simulink model "PID_Controller_Simulink"  (R2023b)
settings: Solver=VariableStepAuto  StartTime=0.0  StopTime=10  RelTol=1e-3
settings Model: Creator=Lenovo  LastModifiedBy=KhyathiB

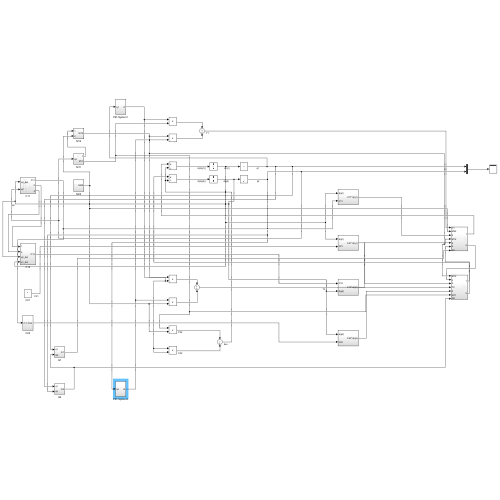
[thumbnail: Simulink's stored preview of the top-level diagram]
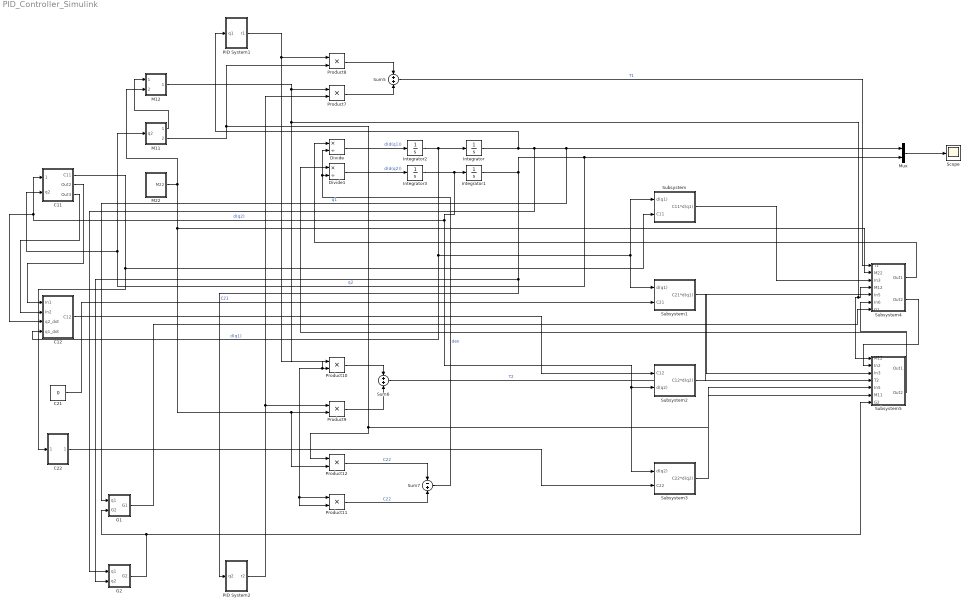
== system PID_Controller_Simulink ==
  C11 : Subsystem
  C12 : Subsystem
  C21 : Constant  Value=0
  C22 : Subsystem
  Divide : Product  Inputs=*/
  Divide1 : Product  Inputs=*/
  G1 : Subsystem
  G2 : Subsystem
  Integrator : Integrator  InitialCondition=0.1
  Integrator1 : Integrator  InitialCondition=0.1
  Integrator2 : Integrator
  Integrator3 : Integrator
  M11 : Subsystem
  M12 : Subsystem
  M22 : Subsystem
  Mux : Mux  Inputs=2
  PID System1 : Subsystem
  PID System2 : Subsystem
  Product{7..12} (6 alike) : Product
  Scope : Scope
  Subsystem : Subsystem
  Subsystem1 : Subsystem
  Subsystem2 : Subsystem
  Subsystem3 : Subsystem
  Subsystem4 : Subsystem
  Subsystem5 : Subsystem
  Sum5 : Sum
  Sum6 : Sum
  Sum7 : Sum  Inputs=-+
  wires:
  Mux/1 -> Scope/1
  Integrator/1 -> G2/1(q1), G1/1(q1), Mux/1, PID System1/1(q1)  "q1"
  Integrator1/1 -> G2/2(q2), PID System2/1(q2), C11/2(q2), M11/1(q2), Mux/2  "q2"
  Integrator2/1 -> Integrator/1, C12/4(q1_dot), Subsystem1/1(d(q1)), Subsystem/1(d(q1))  "d(q1)"
  Integrator3/1 -> Subsystem3/1(d(q2)), Subsystem2/2(d(q2)), C12/3(q2_dot), C11/1(q2_dot), Integrator1/1  "d(q2)"
  Divide1/1 -> Integrator3/1  "d(d(q2))"
  Divide/1 -> Integrator2/1  "d(d(q1))"
  PID System2/1(r2) -> Product7/2, Product9/1
  PID System1/1(r1) -> Product10/1, Product8/1
  Product8/1 -> Sum5/1
  Product7/1 -> Sum5/2
  Product9/1 -> Sum6/2
  Product10/1 -> Sum6/1
  Product12/1 -> Sum7/1  "C22"
  Product11/1 -> Sum7/2  "C22"
  Sum7/1 -> Divide/2, Divide1/2  "den"
  C21/1 -> Subsystem1/2(C21)  "C21"
  Sum5/1 -> Subsystem4/1(T1)  "T1"
  Subsystem/1(C11*d(q1)) -> Subsystem4/3(In3)
  Subsystem2/1(C12*d(q2)) -> Subsystem4/5(In5)
  Subsystem4/1(Out1) -> Divide/1
  Subsystem4/2(Out2) -> Subsystem5/2(In2)
  Subsystem1/1(C21*d(q1)) -> Subsystem5/3(In3)
  Sum6/1 -> Subsystem5/4(T2)  "T2"
  Subsystem3/1(C22*d(q2)) -> Subsystem5/5(In5)
  Subsystem5/1(Out1) -> Divide1/1
  Subsystem5/2(Out2) -> Subsystem4/6(In6)
  M22/1(M22) -> M12/2(In2), Subsystem4/2(M22), Product9/2, Product12/2
  M11/2(M11) -> Product8/2, Product12/1, Subsystem5/6(M11)
  M12/1(M12) -> Product11/1, Product11/2, Product10/2, Subsystem4/4(M12), Subsystem5/1(M12), Product7/1
  M11/1(Out1) -> M12/1(In1)
  C11/1(C11) -> C22/1(C11), Subsystem/2(C11)
  C11/2(Out2) -> C12/1(In1)
  C11/3(Out3) -> C12/2(In2)
  C12/1(C12) -> Subsystem2/1(C12)
  C22/1(C22) -> Subsystem3/2(C22)
  G2/1(G2) -> G1/2(G2), Subsystem5/7(G2)
  G1/1(G1) -> Subsystem4/7(G1)

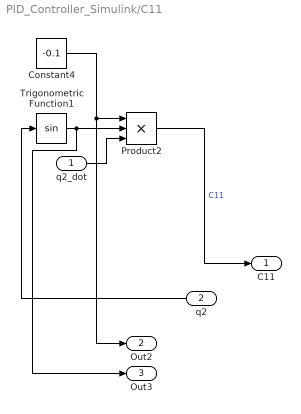
== system PID_Controller_Simulink/C11 ==
  q2_dot : Inport
  q2 : Inport  Port=2
  Constant4 : Constant  Value=-0.1
  Product2 : Product  Inputs=3
  Trigonometric Function1 : Trigonometry
  C11 : Outport
  Out2 : Outport  Port=2
  Out3 : Outport  Port=3
  wires:
  Constant4/1 -> Out2/1, Product2/1
  Trigonometric Function1/1 -> Out3/1, Product2/2
  q2/1 -> Trigonometric Function1/1
  Product2/1 -> C11/1  "C11"
  q2_dot/1 -> Product2/3

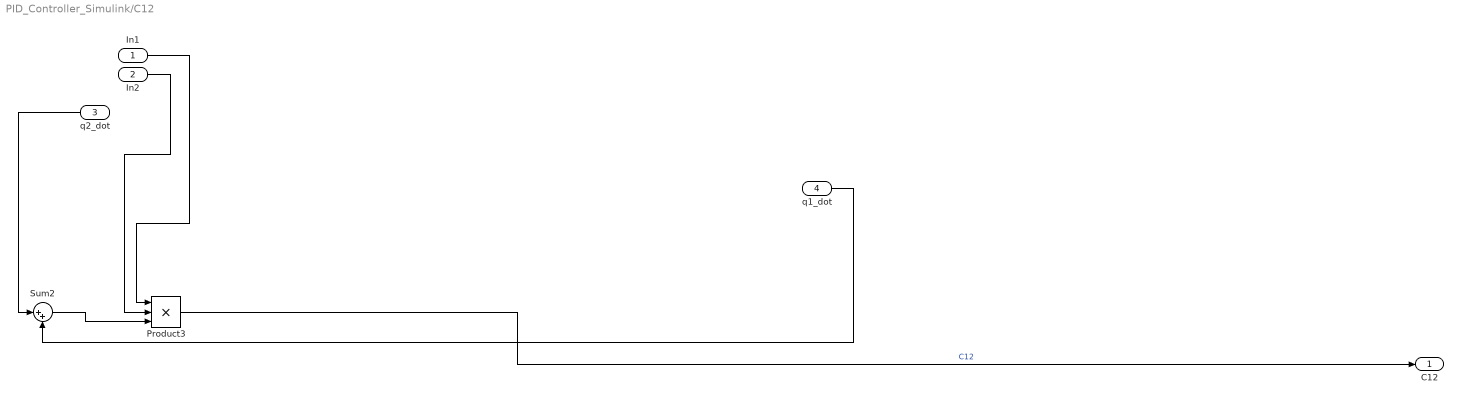
== system PID_Controller_Simulink/C12 ==
  In1 : Inport
  In2 : Inport  Port=2
  q2_dot : Inport  Port=3
  q1_dot : Inport  Port=4
  Product3 : Product  Inputs=3
  Sum2 : Sum  Inputs=|++
  C12 : Outport
  wires:
  In2/1 -> Product3/2
  Sum2/1 -> Product3/3
  q2_dot/1 -> Sum2/1
  q1_dot/1 -> Sum2/2
  Product3/1 -> C12/1  "C12"
  In1/1 -> Product3/1

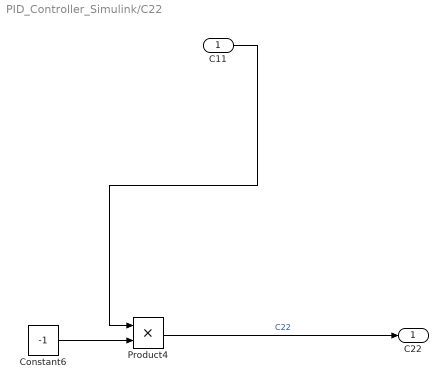
== system PID_Controller_Simulink/C22 ==
  C11 : Inport
  Constant6 : Constant  Value=-1
  Product4 : Product
  C22 : Outport
  wires:
  Constant6/1 -> Product4/2
  Product4/1 -> C22/1  "C22"
  C11/1 -> Product4/1

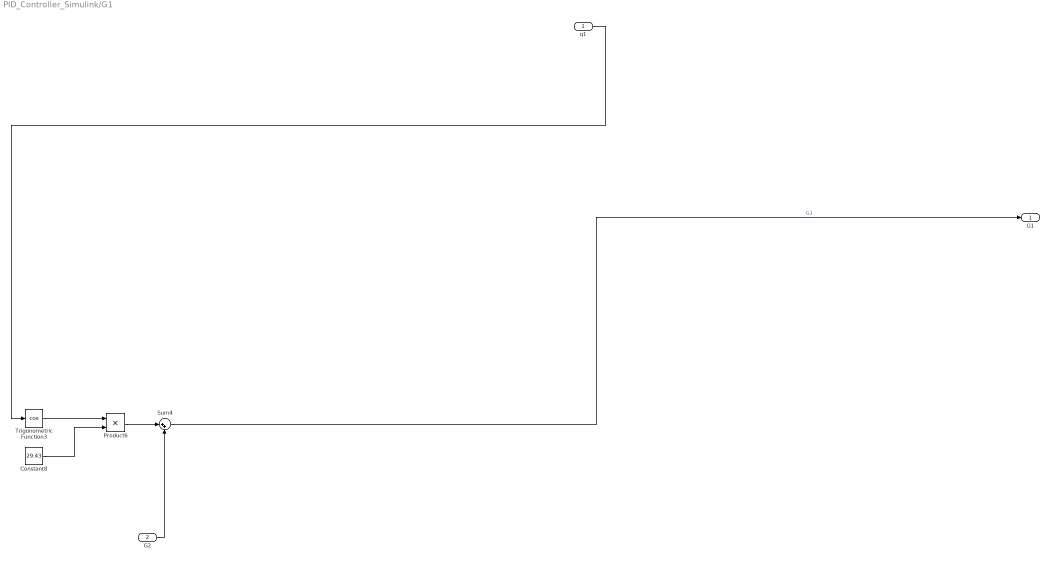
== system PID_Controller_Simulink/G1 ==
  q1 : Inport
  G2 : Inport  Port=2
  Constant8 : Constant  Value=29.43
  Product6 : Product
  Sum4 : Sum  Inputs=|++
  Trigonometric Function3 : Trigonometry  Operator=cos
  G1 : Outport
  wires:
  Sum4/1 -> G1/1  "G1"
  Constant8/1 -> Product6/2
  Product6/1 -> Sum4/1
  G2/1 -> Sum4/2
  Trigonometric Function3/1 -> Product6/1
  q1/1 -> Trigonometric Function3/1

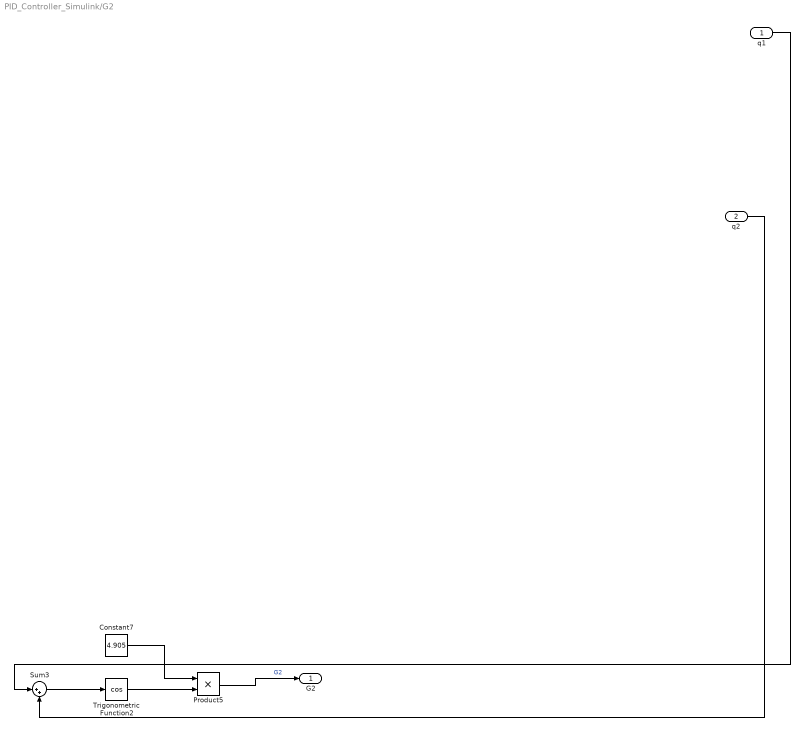
== system PID_Controller_Simulink/G2 ==
  q1 : Inport
  q2 : Inport  Port=2
  Constant7 : Constant  Value=4.905
  Product5 : Product
  Sum3 : Sum  Inputs=|++
  Trigonometric Function2 : Trigonometry  Operator=cos
  G2 : Outport
  wires:
  Constant7/1 -> Product5/1
  Product5/1 -> G2/1  "G2"
  q2/1 -> Sum3/2
  q1/1 -> Sum3/1
  Sum3/1 -> Trigonometric Function2/1
  Trigonometric Function2/1 -> Product5/2

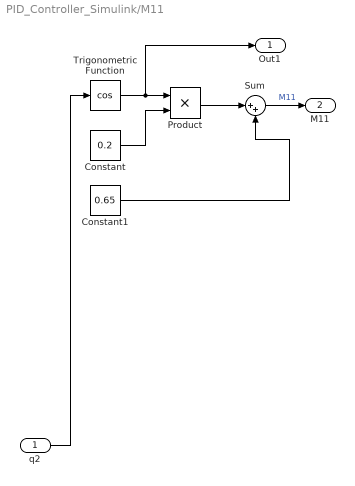
== system PID_Controller_Simulink/M11 ==
  q2 : Inport
  Constant : Constant  Value=0.2
  Constant1 : Constant  Value=0.65
  Product : Product
  Sum : Sum  Inputs=|++
  Trigonometric Function : Trigonometry  Operator=cos
  Out1 : Outport
  M11 : Outport  Port=2
  wires:
  q2/1 -> Trigonometric Function/1
  Trigonometric Function/1 -> Out1/1, Product/1
  Constant/1 -> Product/2
  Sum/1 -> M11/1  "M11"
  Constant1/1 -> Sum/2
  Product/1 -> Sum/1

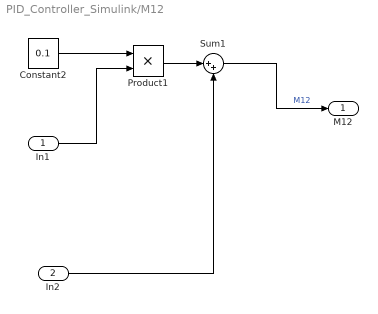
== system PID_Controller_Simulink/M12 ==
  In1 : Inport
  In2 : Inport  Port=2
  Constant2 : Constant  Value=0.1
  Product1 : Product
  Sum1 : Sum  Inputs=|++
  M12 : Outport
  wires:
  Product1/1 -> Sum1/1
  Constant2/1 -> Product1/1
  In1/1 -> Product1/2
  Sum1/1 -> M12/1  "M12"
  In2/1 -> Sum1/2

== system PID_Controller_Simulink/M22 ==
  Constant3 : Constant  Value=0.05
  M22 : Outport
  wires:
  Constant3/1 -> M22/1  "M22"

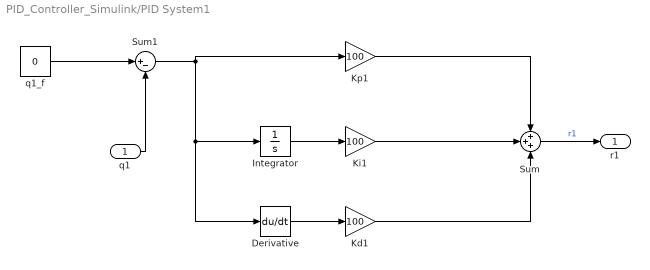
== system PID_Controller_Simulink/PID System1 ==
  q1 : Inport
  Derivative : Derivative
  Integrator : Integrator
  Kd1 : Gain  Gain=100
  Ki1 : Gain  Gain=100
  Kp1 : Gain  Gain=100
  Sum : Sum  Inputs=+++
  Sum1 : Sum  Inputs=|+-
  q1_f : Constant  Value=0
  r1 : Outport
  wires:
  Integrator/1 -> Ki1/1
  Sum1/1 -> Derivative/1, Integrator/1, Kp1/1
  Kp1/1 -> Sum/1
  Kd1/1 -> Sum/3
  Derivative/1 -> Kd1/1
  q1/1 -> Sum1/2
  Ki1/1 -> Sum/2
  q1_f/1 -> Sum1/1
  Sum/1 -> r1/1  "r1"

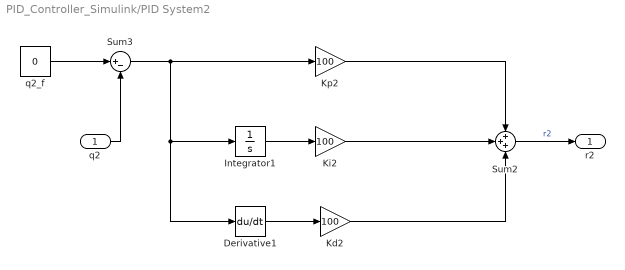
== system PID_Controller_Simulink/PID System2 ==
  q2 : Inport
  Derivative1 : Derivative
  Integrator1 : Integrator
  Kd2 : Gain  Gain=100
  Ki2 : Gain  Gain=100
  Kp2 : Gain  Gain=100
  Sum2 : Sum  Inputs=+++
  Sum3 : Sum  Inputs=|+-
  q2_f : Constant  Value=0
  r2 : Outport
  wires:
  Ki2/1 -> Sum2/2
  Sum3/1 -> Derivative1/1, Integrator1/1, Kp2/1
  q2_f/1 -> Sum3/1
  Kd2/1 -> Sum2/3
  Derivative1/1 -> Kd2/1
  Integrator1/1 -> Ki2/1
  q2/1 -> Sum3/2
  Kp2/1 -> Sum2/1
  Sum2/1 -> r2/1  "r2"

== system PID_Controller_Simulink/Subsystem ==
  d(q1) : Inport
  C11 : Inport  Port=2
  Product13 : Product
  C11*d(q1) : Outport
  wires:
  Product13/1 -> C11*d(q1)/1  "C11*q1_dot"
  d(q1)/1 -> Product13/1
  C11/1 -> Product13/2

== system PID_Controller_Simulink/Subsystem1 ==
  d(q1) : Inport
  C21 : Inport  Port=2
  Product14 : Product
  C21*d(q1) : Outport
  wires:
  d(q1)/1 -> Product14/1
  C21/1 -> Product14/2
  Product14/1 -> C21*d(q1)/1  "C21*q1_dot"

== system PID_Controller_Simulink/Subsystem2 ==
  C12 : Inport
  d(q2) : Inport  Port=2
  Product15 : Product
  C12*d(q2) : Outport
  wires:
  d(q2)/1 -> Product15/2
  C12/1 -> Product15/1
  Product15/1 -> C12*d(q2)/1  "C12*q2_dot"

== system PID_Controller_Simulink/Subsystem3 ==
  d(q2) : Inport
  C22 : Inport  Port=2
  Product16 : Product
  C22*d(q2) : Outport
  wires:
  Product16/1 -> C22*d(q2)/1  "C22*q2_dot"
  d(q2)/1 -> Product16/1
  C22/1 -> Product16/2

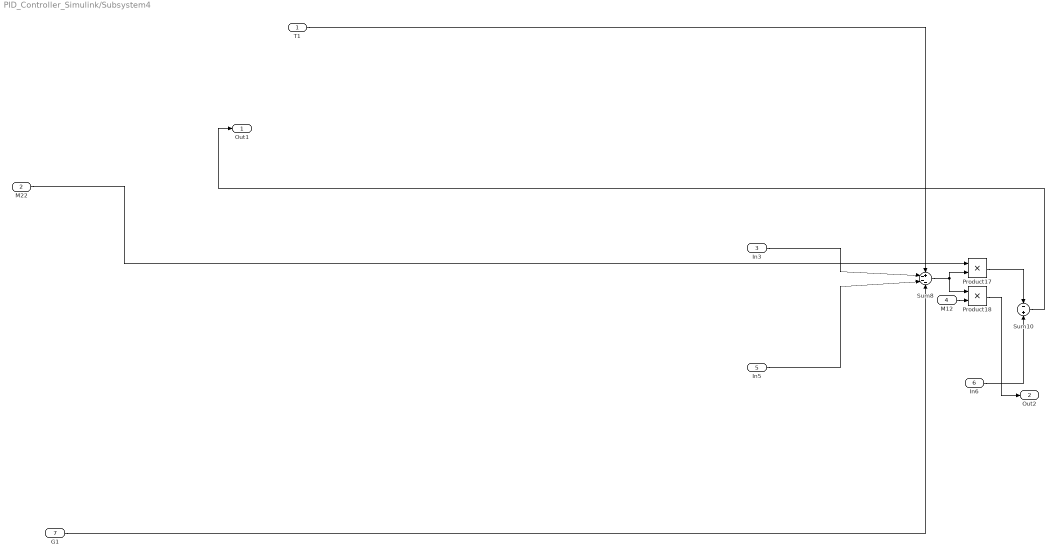
== system PID_Controller_Simulink/Subsystem4 ==
  T1 : Inport
  M22 : Inport  Port=2
  In3 : Inport  Port=3
  M12 : Inport  Port=4
  In5 : Inport  Port=5
  In6 : Inport  Port=6
  G1 : Inport  Port=7
  Product17 : Product
  Product18 : Product
  Sum10 : Sum  Inputs=-+
  Sum8 : Sum  Inputs=+---
  Out1 : Outport
  Out2 : Outport  Port=2
  wires:
  Product18/1 -> Out2/1
  G1/1 -> Sum8/4
  T1/1 -> Sum8/1
  In6/1 -> Sum10/2
  Sum8/1 -> Product18/1, Product17/2
  Product17/1 -> Sum10/1
  In3/1 -> Sum8/2
  Sum10/1 -> Out1/1
  M22/1 -> Product17/1
  In5/1 -> Sum8/3
  M12/1 -> Product18/2

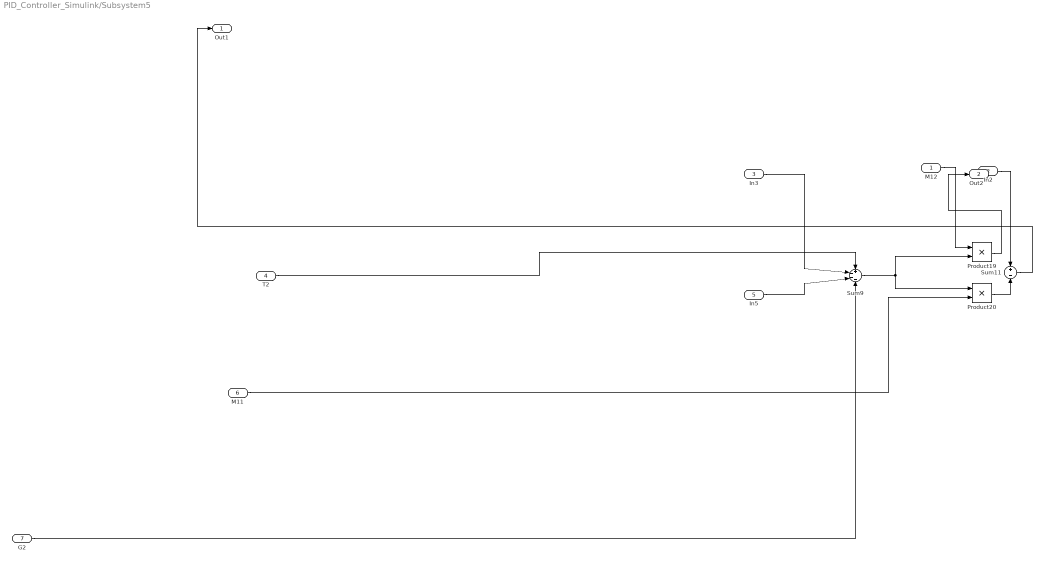
== system PID_Controller_Simulink/Subsystem5 ==
  M12 : Inport
  In2 : Inport  Port=2
  In3 : Inport  Port=3
  T2 : Inport  Port=4
  In5 : Inport  Port=5
  M11 : Inport  Port=6
  G2 : Inport  Port=7
  Product19 : Product
  Product20 : Product
  Sum11 : Sum  Inputs=+-
  Sum9 : Sum  Inputs=+---
  Out1 : Outport
  Out2 : Outport  Port=2
  wires:
  In3/1 -> Sum9/2
  Product19/1 -> Out2/1
  G2/1 -> Sum9/4
  Sum9/1 -> Product19/2, Product20/1
  In5/1 -> Sum9/3
  In2/1 -> Sum11/1
  M12/1 -> Product19/1
  Sum11/1 -> Out1/1
  M11/1 -> Product20/2
  Product20/1 -> Sum11/2
  T2/1 -> Sum9/1
